simulink model "SImulacao_sistema_tanques"  (R2021a)
settings: Solver=VariableStepAuto  StartTime=0.0  StopTime=100.0  RelTol=1e-3
settings Model: Creator=Pedro  LastModifiedBy=Pedro

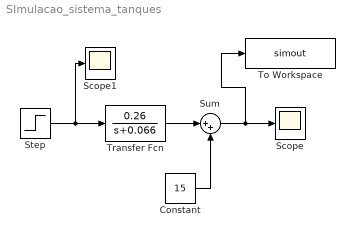
== system SImulacao_sistema_tanques ==
  Constant : Constant  Value=15
  Scope : Scope
  Scope1 : Scope
  Step : Step  Time=0  Before=0.763  After=0.763  SampleTime=0
  Sum : Sum  Inputs=|++
  To Workspace : ToWorkspace  VariableName=simout  SaveFormat=Timeseries  SampleTime=-1
  Transfer Fcn : TransferFcn  Numerator=[0.26]  Denominator=[1 0.066]
  wires:
  Step/1 -> Scope1/1, Transfer Fcn/1
  Transfer Fcn/1 -> Sum/1
  Constant/1 -> Sum/2
  Sum/1 -> To Workspace/1, Scope/1
